simulink model "uz_SVPWM_6ph"  (R2024a)
settings: Solver=FixedStepDiscrete  StartTime=0.0  StopTime=0.0004  RelTol=1e-3
values from neighbouring files (symbols this model uses):
  f_FPGA_clk = 100e6    (= 100000000)    [Init_IP_Core.m]
  T_FPGA_clk = 1/f_FPGA_clk    (= 1e-08)    [Init_IP_Core.m]
libraries: hdlsllib x7, simulink x1
settings Model: DataTypeOverride=Off  Creator=josef  LastModifiedBy=josef
settings SolverCC: AlgebraicLoopSolver=TrustRegion
settings DataIOCC: LimitDataPoints=on  SaveOutput=off  SaveTime=off
settings OptimizationCC: BlockReduction=off  ConditionallyExecuteInputs=off  DefaultParameterBehavior=Inlined  LifeSpan=inf
settings DebuggingCC: AlgebraicLoopMsg=error  SingleTaskRateTransMsg=error  UnconnectedInputMsg=warning  UnconnectedOutputMsg=warning  UnconnectedLineMsg=warning  AllowSymbolicDim=off  StrictBusMsg=ErrorOnBusTreatedAsVector  SFUnexpectedBacktrackingDiag=warning  SFNoUnconditionalDefaultTransitionDiag=warning  SFExecutionAtInitializationDiag=none  ArithmeticOperatorsInVariantConditions=warning
settings HardwareCC: ProdBitPerPointer=32  ProdBitPerSizeT=32  ProdBitPerPtrDiffT=32  ProdLargestAtomicFloat=None  ProdIntDivRoundTo=Undefined  ProdEndianess=Unspecified  ProdWordSize=32  ProdHWDeviceType=ASIC/FPGA->ASIC/FPGA  ProdEqTarget=off
settings ModelReferenceCC: EnableRefExpFcnMdlSchedulingChecks=on
settings SFSimCC: SimUseLocalCustomCode=off  CustomCodeUndefinedFunction=UseInterfaceOnly
settings RTWCC: RTWUseLocalCustomCode=off  GPUComputeCapability=3.5
settings CodeAppCC: StateflowObjectComments=on
settings GRTTargetCC: TargetLangStandard=C89/C90 (ANSI)
settings ConfigComp: CovScope=ReferencedModels  CovMetricSettings=dw  CovSaveCumulativeToWorkspaceVar=on  CovSaveSingleToWorkspaceVar=on  CovExternalEMLEnable=off  CovSFcnEnable=off

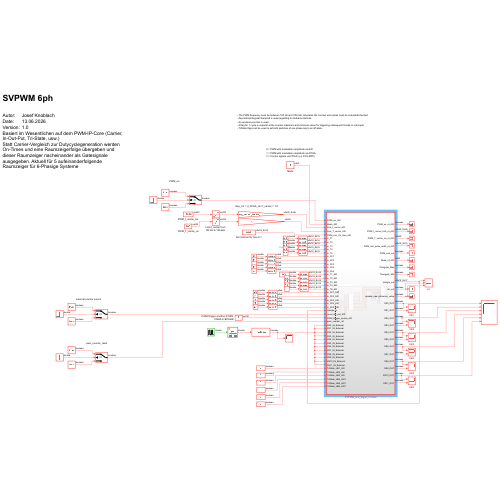
[thumbnail: Simulink's stored preview of the top-level diagram]
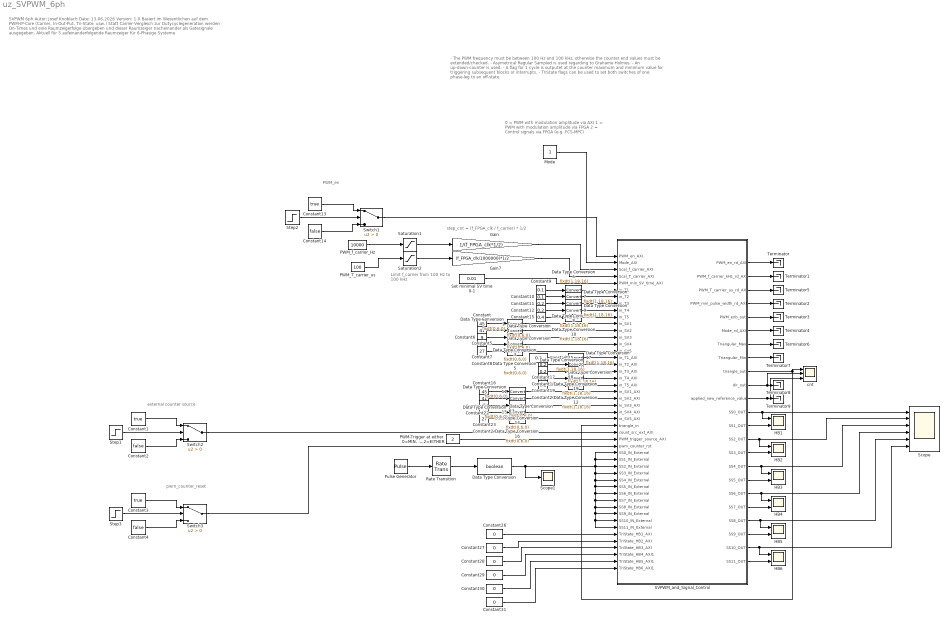
== system uz_SVPWM_6ph ==
  note: PWM_en
  note: Limit f_carrier from
      | 100 Hz to 100 kHz
  note: - The PWM frequency must be between 100 Hz and 100 kHz, otherwise the counter end values must be extended/checked.
      | - Asymetrical Regular Sampled is used regarding to Grahame Holmes.
      | - An up-down-counter is used.
      | - A flag for 1 cycle is outputet at the counter maximum and minimum value for triggering subsequent blocks or interrupts.
      | - TriState flags can be used to set both switches of one phase-leg to an off-state.
  note: SVPWM 6ph
      |
      | Autor: Josef Knoblach
      | Date: 13.06.2026
      | Version: 1.0
      | Basiert im Wesentlichen auf dem PWM-IP-Core (Carrier, In-Out-Put, Tri-State, usw.)
      | Statt Carrier-Vergleich zur Dutycyclegeneration werden On-Times und eine Raumzeigerfolge übergeben und dieser Raumzeiger nacheinander als Gatesignale ausgegeben. Aktuell für 5 aufeinanderfolgende Raumzeiger für 6-Phasige Systeme
  note: step_cnt = (f_FPGA_clk / f_carrier) * 1/2
  note: 0 = PWM with modulation amplitude via AXI
      | 1 = PWM with modulation amplitude via FPGA
      | 2 = Control signals via FPGA (e.g. FCS-MPC)
  note: external counter source
  note: pwm_counter_reset
  Constant : Constant  Value=45  SampleTime=T_FPGA_clk
  Constant1 : Constant  Value=true  SampleTime=T_FPGA_clk
  Constant10 : Constant  Value=0.1  SampleTime=T_FPGA_clk
  Constant{11..12,17..18,20} (5 alike) : Constant  Value=0.2  SampleTime=T_FPGA_clk
  Constant13 : Constant  Value=true  SampleTime=T_FPGA_clk
  Constant14 : Constant  Value=false  SampleTime=T_FPGA_clk
  Constant15 : Constant  Value=0.4  SampleTime=T_FPGA_clk
  Constant16 : Constant  Value=45  SampleTime=T_FPGA_clk
  Constant19 : Constant  Value=0.1  SampleTime=T_FPGA_clk
  Constant2 : Constant  Value=false  SampleTime=T_FPGA_clk
  Constant21 : Constant  Value=41  SampleTime=T_FPGA_clk
  Constant22 : Constant  Value=9  SampleTime=T_FPGA_clk
  Constant23 : Constant  Value=11  SampleTime=T_FPGA_clk
  Constant24 : Constant  Value=27  SampleTime=T_FPGA_clk
  Constant25 : Constant  Value=0.3  SampleTime=T_FPGA_clk
  Constant{26..31} (6 alike) : Constant  Value=0  OutDataTypeStr=boolean  SampleTime=T_FPGA_clk
  Constant3 : Constant  Value=true  SampleTime=T_FPGA_clk
  Constant4 : Constant  Value=false  SampleTime=T_FPGA_clk
  Constant5 : Constant  Value=41  SampleTime=T_FPGA_clk
  Constant6 : Constant  Value=9  SampleTime=T_FPGA_clk
  Constant7 : Constant  Value=11  SampleTime=T_FPGA_clk
  Constant8 : Constant  Value=27  SampleTime=T_FPGA_clk
  Constant9 : Constant  Value=0.1  SampleTime=T_FPGA_clk
  Data Type Conversion : DataTypeConversion  OutDataTypeStr=boolean  SaturateOnIntegerOverflow=off  RndMeth=Floor
  Data Type Conversion{1..5,11,13..16} (10 alike) : DataTypeConversion  OutDataTypeStr=fixdt(0,6,0)  SaturateOnIntegerOverflow=off  RndMeth=Floor
  Data Type Conversion{6..10,12,17..20} (10 alike) : DataTypeConversion  OutDataTypeStr=fixdt(1,18,16)  SaturateOnIntegerOverflow=off  RndMeth=Floor
  Gain : Gain  Gain=1/(f_FPGA_clk*1/2)  OutDataTypeStr=fixdt(0,25,26)
  Gain7 : Gain  Gain=(f_FPGA_clk/1000000)*1/2  OutDataTypeStr=fixdt(0,25,0)
  HB{1..6} (6 alike) : Scope  NumInputPorts=2
  Mode : Constant  OutDataTypeStr=fixdt(0,2,0)  SampleTime=T_FPGA_clk
  "PWM-Trigger at either 0=MIN, 1=MAX,2=EITHER" : Constant  Value=2  OutDataTypeStr=uint32  SampleTime=T_FPGA_clk
  PWM_T_carrier_us : Constant  Value=100  OutDataTypeStr=uint32  SampleTime=T_FPGA_clk
  PWM_f_carrier_Hz : Constant  Value=10000  OutDataTypeStr=uint32  SampleTime=T_FPGA_clk
  Pulse Generator : DiscretePulseGenerator  PulseType=Time based  Period=0.0001  PulseWidth=5
  Rate Transition : RateTransition  OutPortSampleTime=T_FPGA_clk
  SVPWM_and_Signal_Control : Subsystem  TreatAsAtomicUnit=on
  Saturation1 : Saturate  UpperLimit=100000  LowerLimit=100
  Saturation2 : Saturate  UpperLimit=10000  LowerLimit=10
  Scope : Scope  NumInputPorts=6
  Scope1 : Scope
  Set minimal SV time 0-1 : Constant  Value=0.01  OutDataTypeStr=fixdt(1,18,16)  SampleTime=T_FPGA_clk
  Step1 : Step  Time=0.002  After=0  SampleTime=T_FPGA_clk
  Step2 : Step  Time=0.002  Before=1  SampleTime=T_FPGA_clk
  Step3 : Step  Time=0.00025  SampleTime=T_FPGA_clk
  Switch1 : Switch  Criteria=u2 > Threshold  SaturateOnIntegerOverflow=off  InputSameDT=off
  Switch2 : Switch  Criteria=u2 > Threshold  SaturateOnIntegerOverflow=off  InputSameDT=off
  Switch3 : Switch  Criteria=u2 > Threshold  SaturateOnIntegerOverflow=off  InputSameDT=off
  Terminator{,1..9} (10 alike) : Terminator
  cnt : Scope  NumInputPorts=3
  wires:
  SVPWM_and_Signal_Control/9(triangle_out) -> SVPWM_and_Signal_Control/26(triangle_in), cnt/1
  Constant3/1 -> Switch3/1
  Pulse Generator/1 -> Rate Transition/1
  SVPWM_and_Signal_Control/11(applied_new_reference_value) -> cnt/3, Terminator9/1
  Constant4/1 -> Switch3/3
  Switch1/1 -> SVPWM_and_Signal_Control/1(PWM_en_AXI)
  SVPWM_and_Signal_Control/1(PWM_en_rd_AXI) -> Terminator/1
  Step3/1 -> Switch3/2
  "PWM-Trigger at either 0=MIN, 1=MAX,2=EITHER"/1 -> SVPWM_and_Signal_Control/28(PWM_trigger_source_AXI)
  SVPWM_and_Signal_Control/3(PWM_T_carrier_us_rd_AXI) -> Terminator5/1
  Switch3/1 -> SVPWM_and_Signal_Control/29(pwm_counter_rst)
  Switch2/1 -> SVPWM_and_Signal_Control/27(count_src_ext_AXI)
  SVPWM_and_Signal_Control/4(PWM_min_pulse_width_rd_AXI) -> Terminator2/1
  Rate Transition/1 -> Data Type Conversion/1
  PWM_T_carrier_us/1 -> Saturation2/1
  Step1/1 -> Switch2/2
  Saturation2/1 -> Gain7/1
  Saturation1/1 -> Gain/1
  Constant2/1 -> Switch2/3
  Constant14/1 -> Switch1/3
  SVPWM_and_Signal_Control/10(dir_out) -> cnt/2, Terminator8/1
  Constant1/1 -> Switch2/1
  SVPWM_and_Signal_Control/7(Triangular_Max) -> Terminator6/1
  SVPWM_and_Signal_Control/2(PWM_f_carrier_kHz_rd_AXI) -> Terminator1/1
  SVPWM_and_Signal_Control/5(PWM_enb_out) -> Terminator3/1
  Gain7/1 -> SVPWM_and_Signal_Control/4(Scal_T_carrier_AXI)
  SVPWM_and_Signal_Control/6(Mode_rd_AXI) -> Terminator4/1
  Gain/1 -> SVPWM_and_Signal_Control/3(Scal_f_carrier_AXI)
  SVPWM_and_Signal_Control/8(Triangular_Min) -> Terminator7/1
  Step2/1 -> Switch1/2
  Set minimal SV time 0-1/1 -> SVPWM_and_Signal_Control/5(PWM_min_SV_time_AXI)
  Mode/1 -> SVPWM_and_Signal_Control/2(Mode_AXI)
  PWM_f_carrier_Hz/1 -> Saturation1/1
  Constant13/1 -> Switch1/1
  Data Type Conversion5/1 -> SVPWM_and_Signal_Control/15(in_SV5)
  Data Type Conversion4/1 -> SVPWM_and_Signal_Control/14(in_SV4)
  Data Type Conversion3/1 -> SVPWM_and_Signal_Control/13(in_SV3)
  Data Type Conversion2/1 -> SVPWM_and_Signal_Control/12(in_SV2)
  Data Type Conversion1/1 -> SVPWM_and_Signal_Control/11(in_SV1)
  Constant/1 -> Data Type Conversion1/1
  Constant8/1 -> Data Type Conversion5/1
  Constant7/1 -> Data Type Conversion4/1
  Constant6/1 -> Data Type Conversion3/1
  Constant5/1 -> Data Type Conversion2/1
  Constant10/1 -> Data Type Conversion7/1
  Constant11/1 -> Data Type Conversion8/1
  Constant12/1 -> Data Type Conversion9/1
  Constant15/1 -> Data Type Conversion10/1
  Constant9/1 -> Data Type Conversion6/1
  Data Type Conversion6/1 -> SVPWM_and_Signal_Control/6(in_T1)
  Data Type Conversion10/1 -> SVPWM_and_Signal_Control/10(in_T5)
  Data Type Conversion9/1 -> SVPWM_and_Signal_Control/9(in_T4)
  Data Type Conversion8/1 -> SVPWM_and_Signal_Control/8(in_T3)
  Data Type Conversion7/1 -> SVPWM_and_Signal_Control/7(in_T2)
  Data Type Conversion18/1 -> SVPWM_and_Signal_Control/17(in_T2_AXI)
  Data Type Conversion19/1 -> SVPWM_and_Signal_Control/18(in_T3_AXI)
  Data Type Conversion20/1 -> SVPWM_and_Signal_Control/19(in_T4_AXI)
  Data Type Conversion12/1 -> SVPWM_and_Signal_Control/20(in_T5_AXI)
  Data Type Conversion17/1 -> SVPWM_and_Signal_Control/16(in_T1_AXI)
  Constant25/1 -> Data Type Conversion17/1
  Constant20/1 -> Data Type Conversion12/1
  Constant19/1 -> Data Type Conversion20/1
  Constant18/1 -> Data Type Conversion19/1
  Constant17/1 -> Data Type Conversion18/1
  Constant21/1 -> Data Type Conversion13/1
  Constant22/1 -> Data Type Conversion14/1
  Constant23/1 -> Data Type Conversion15/1
  Constant24/1 -> Data Type Conversion16/1
  Constant16/1 -> Data Type Conversion11/1
  Data Type Conversion11/1 -> SVPWM_and_Signal_Control/21(in_SV1_AXI)
  Data Type Conversion13/1 -> SVPWM_and_Signal_Control/22(in_SV2_AXI)
  Data Type Conversion14/1 -> SVPWM_and_Signal_Control/23(in_SV3_AXI)
  Data Type Conversion15/1 -> SVPWM_and_Signal_Control/24(in_SV4_AXI)
  Data Type Conversion16/1 -> SVPWM_and_Signal_Control/25(in_SV5_AXI)
  Data Type Conversion/1 -> Scope1/1, SVPWM_and_Signal_Control/41(SS11_IN_External), SVPWM_and_Signal_Control/40(SS10_IN_External), SVPWM_and_Signal_Control/39(SS9_IN_External), SVPWM_and_Signal_Control/38(SS8_IN_External), SVPWM_and_Signal_Control/37(SS7_IN_External), SVPWM_and_Signal_Control/36(SS6_IN_External), SVPWM_and_Signal_Control/35(SS5_IN_External), SVPWM_and_Signal_Control/34(SS4_IN_External), SVPWM_and_Signal_Control/33(SS3_IN_External), SVPWM_and_Signal_Control/32(SS2_IN_External), SVPWM_and_Signal_Control/31(SS1_IN_External), SVPWM_and_Signal_Control/30(SS0_IN_External)
  Constant26/1 -> SVPWM_and_Signal_Control/42(TriState_HB1_AXI)
  Constant27/1 -> SVPWM_and_Signal_Control/43(TriState_HB2_AXI)
  Constant28/1 -> SVPWM_and_Signal_Control/44(TriState_HB3_AXI)
  Constant29/1 -> SVPWM_and_Signal_Control/45(TriState_HB4_AXI1)
  Constant30/1 -> SVPWM_and_Signal_Control/46(TriState_HB5_AXI1)
  Constant31/1 -> SVPWM_and_Signal_Control/47(TriState_HB6_AXI1)
  SVPWM_and_Signal_Control/12(SS0_OUT) -> HB1/1, Scope/1
  SVPWM_and_Signal_Control/14(SS2_OUT) -> HB2/1, Scope/2
  SVPWM_and_Signal_Control/16(SS4_OUT) -> HB3/1, Scope/3
  SVPWM_and_Signal_Control/18(SS6_OUT) -> HB4/1, Scope/4
  SVPWM_and_Signal_Control/20(SS8_OUT) -> HB5/1, Scope/5
  SVPWM_and_Signal_Control/22(SS10_OUT) -> HB6/1, Scope/6
  SVPWM_and_Signal_Control/13(SS1_OUT) -> HB1/2
  SVPWM_and_Signal_Control/23(SS11_OUT) -> HB6/2
  SVPWM_and_Signal_Control/21(SS9_OUT) -> HB5/2
  SVPWM_and_Signal_Control/19(SS7_OUT) -> HB4/2
  SVPWM_and_Signal_Control/17(SS5_OUT) -> HB3/2
  SVPWM_and_Signal_Control/15(SS3_OUT) -> HB2/2

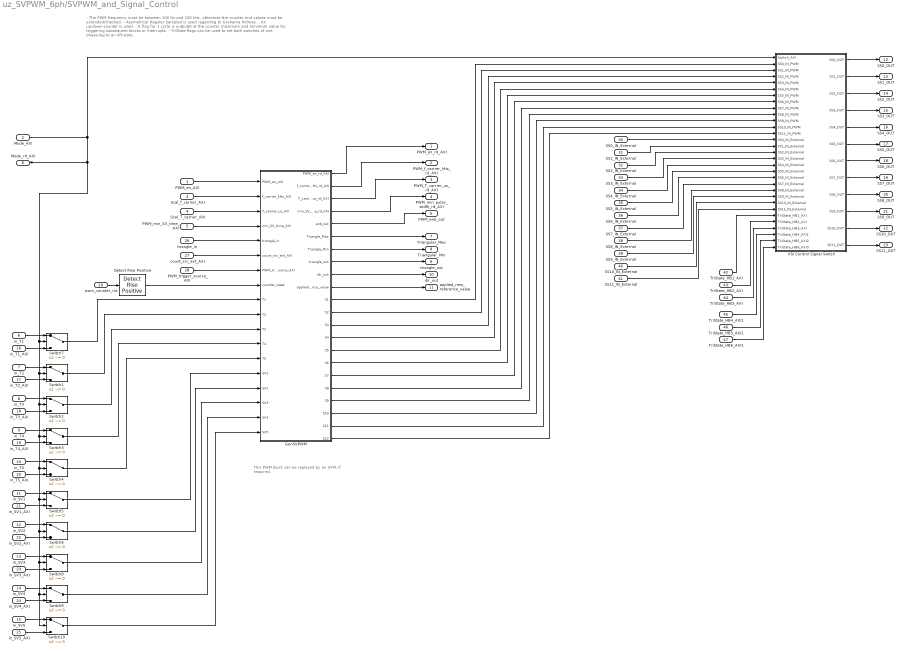
== system uz_SVPWM_6ph/SVPWM_and_Signal_Control ==
  note: This PWM block can be replaced by an SVM,
      | if required.
  note: - The PWM frequency must be between 100 Hz and 100 kHz, otherwise the counter end values must be extended/checked.
      | - Asymetrical Regular Sampled is used regarding to Grahame Holmes.
      | - An up-down-counter is used.
      | - A flag for 1 cycle is outputet at the counter maximum and minimum value for triggering subsequent blocks or interrupts.
      | - TriState flags can be used to set both switches of one phase-leg to an off-state.
  PWM_en_AXI : Inport
  Mode_AXI : Inport  Port=2
  Scal_f_carrier_AXI : Inport  Port=3
  Scal_T_carrier_AXI : Inport  Port=4
  PWM_min_SV_time_AXI : Inport  Port=5
  in_T1 : Inport  Port=6
  in_T2 : Inport  Port=7
  in_T3 : Inport  Port=8
  in_T4 : Inport  Port=9
  in_T5 : Inport  Port=10
  in_SV1 : Inport  Port=11
  in_SV2 : Inport  Port=12
  in_SV3 : Inport  Port=13
  in_SV4 : Inport  Port=14
  in_SV5 : Inport  Port=15
  in_T1_AXI : Inport  Port=16
  in_T2_AXI : Inport  Port=17
  in_T3_AXI : Inport  Port=18
  in_T4_AXI : Inport  Port=19
  in_T5_AXI : Inport  Port=20
  in_SV1_AXI : Inport  Port=21
  in_SV2_AXI : Inport  Port=22
  in_SV3_AXI : Inport  Port=23
  in_SV4_AXI : Inport  Port=24
  in_SV5_AXI : Inport  Port=25
  triangle_in : Inport  Port=26
  count_src_ext_AXI : Inport  Port=27
  PWM_trigger_source_AXI : Inport  Port=28
  pwm_counter_rst : Inport  Port=29
  SS0_IN_External : Inport  Port=30
  SS1_IN_External : Inport  Port=31
  SS2_IN_External : Inport  Port=32
  SS3_IN_External : Inport  Port=33
  SS4_IN_External : Inport  Port=34
  SS5_IN_External : Inport  Port=35
  SS6_IN_External : Inport  Port=36
  SS7_IN_External : Inport  Port=37
  SS8_IN_External : Inport  Port=38
  SS9_IN_External : Inport  Port=39
  SS10_IN_External : Inport  Port=40
  SS11_IN_External : Inport  Port=41
  TriState_HB1_AXI : Inport  Port=42
  TriState_HB2_AXI : Inport  Port=43
  TriState_HB3_AXI : Inport  Port=44
  TriState_HB4_AXI1 : Inport  Port=45
  TriState_HB5_AXI1 : Inport  Port=46
  TriState_HB6_AXI1 : Inport  Port=47
  Detect Rise Positive : simulink/Logic and Bit Operations/Detect Rise Positive  vinit=0  OutDataTypeStr=boolean
  GenSVPWM : Subsystem  TreatAsAtomicUnit=on
  Switch{1..10} (10 alike) : Switch  Criteria=u2 ~= 0  SaturateOnIntegerOverflow=off  InputSameDT=off
  VSI Control Signal Switch : Subsystem
  PWM_en_rd_AXI : Outport  VectorParamsAs1DForOutWhenUnconnected=off
  PWM_f_carrier_kHz_rd_AXI : Outport  Port=2  VectorParamsAs1DForOutWhenUnconnected=off
  PWM_T_carrier_us_rd_AXI : Outport  Port=3  VectorParamsAs1DForOutWhenUnconnected=off
  PWM_min_pulse_width_rd_AXI : Outport  Port=4  VectorParamsAs1DForOutWhenUnconnected=off
  PWM_enb_out : Outport  Port=5  VectorParamsAs1DForOutWhenUnconnected=off
  Mode_rd_AXI : Outport  Port=6  VectorParamsAs1DForOutWhenUnconnected=off
  Triangular_Max : Outport  Port=7  VectorParamsAs1DForOutWhenUnconnected=off
  Triangular_Min : Outport  Port=8  VectorParamsAs1DForOutWhenUnconnected=off
  triangle_out : Outport  Port=9  VectorParamsAs1DForOutWhenUnconnected=off
  dir_out : Outport  Port=10  VectorParamsAs1DForOutWhenUnconnected=off
  applied_new_reference_value : Outport  Port=11  VectorParamsAs1DForOutWhenUnconnected=off
  SS0_OUT : Outport  Port=12  VectorParamsAs1DForOutWhenUnconnected=off
  SS1_OUT : Outport  Port=13  VectorParamsAs1DForOutWhenUnconnected=off
  SS2_OUT : Outport  Port=14  VectorParamsAs1DForOutWhenUnconnected=off
  SS3_OUT : Outport  Port=15  VectorParamsAs1DForOutWhenUnconnected=off
  SS4_OUT : Outport  Port=16  VectorParamsAs1DForOutWhenUnconnected=off
  SS5_OUT : Outport  Port=17  VectorParamsAs1DForOutWhenUnconnected=off
  SS6_OUT : Outport  Port=18  VectorParamsAs1DForOutWhenUnconnected=off
  SS7_OUT : Outport  Port=19  VectorParamsAs1DForOutWhenUnconnected=off
  SS8_OUT : Outport  Port=20  VectorParamsAs1DForOutWhenUnconnected=off
  SS9_OUT : Outport  Port=21  VectorParamsAs1DForOutWhenUnconnected=off
  SS10_OUT : Outport  Port=22  VectorParamsAs1DForOutWhenUnconnected=off
  SS11_OUT : Outport  Port=23  VectorParamsAs1DForOutWhenUnconnected=off
  wires:
  Scal_f_carrier_AXI/1 -> GenSVPWM/2(f_carrier_kHz_AXI)
  GenSVPWM/5(enb_out) -> PWM_enb_out/1
  PWM_en_AXI/1 -> GenSVPWM/1(PWM_en_AXI)
  PWM_min_SV_time_AXI/1 -> GenSVPWM/4(min_SV_time_AXI)
  in_T1_AXI/1 -> Switch7/3
  in_T1/1 -> Switch7/1
  GenSVPWM/1(PWM_en_rd_AXI) -> PWM_en_rd_AXI/1
  GenSVPWM/2(f_carrier_kHz_rd_AXI) -> PWM_f_carrier_kHz_rd_AXI/1
  GenSVPWM/4(min_SV_time_rd_AXI) -> PWM_min_pulse_width_rd_AXI/1
  GenSVPWM/3(T_carrier_us_rd_AXI) -> PWM_T_carrier_us_rd_AXI/1
  Scal_T_carrier_AXI/1 -> GenSVPWM/3(T_carrier_us_AXI)
  GenSVPWM/6(Triangle_Max) -> Triangular_Max/1
  GenSVPWM/7(Triangle_Min) -> Triangular_Min/1
  triangle_in/1 -> GenSVPWM/5(triangle_in)
  GenSVPWM/8(triangle_out) -> triangle_out/1
  GenSVPWM/9(dir_out) -> dir_out/1
  count_src_ext_AXI/1 -> GenSVPWM/6(count_src_ext_AXI)
  PWM_trigger_source_AXI/1 -> GenSVPWM/7(PWM_trigger_source_AXI)
  GenSVPWM/10(applied_new_reference_value) -> applied_new_reference_value/1
  Detect Rise Positive/1 -> GenSVPWM/8(counter_reset)
  pwm_counter_rst/1 -> Detect Rise Positive/1
  VSI Control Signal Switch/8(SS7_OUT) -> SS7_OUT/1
  SS10_IN_External/1 -> VSI Control Signal Switch/24(SS10_IN_External)
  SS8_IN_External/1 -> VSI Control Signal Switch/22(SS8_IN_External)
  SS6_IN_External/1 -> VSI Control Signal Switch/20(SS6_IN_External)
  TriState_HB4_AXI1/1 -> VSI Control Signal Switch/29(TriState_HB4_AXI1)
  TriState_HB2_AXI/1 -> VSI Control Signal Switch/27(TriState_HB2_AXI)
  SS9_IN_External/1 -> VSI Control Signal Switch/23(SS9_IN_External)
  TriState_HB3_AXI/1 -> VSI Control Signal Switch/28(TriState_HB3_AXI)
  VSI Control Signal Switch/10(SS9_OUT) -> SS9_OUT/1
  TriState_HB1_AXI/1 -> VSI Control Signal Switch/26(TriState_HB1_AXI)
  VSI Control Signal Switch/5(SS4_OUT) -> SS4_OUT/1
  VSI Control Signal Switch/1(SS0_OUT) -> SS0_OUT/1
  SS7_IN_External/1 -> VSI Control Signal Switch/21(SS7_IN_External)
  VSI Control Signal Switch/6(SS5_OUT) -> SS5_OUT/1
  SS1_IN_External/1 -> VSI Control Signal Switch/15(SS1_IN_External)
  SS4_IN_External/1 -> VSI Control Signal Switch/18(SS4_IN_External)
  SS3_IN_External/1 -> VSI Control Signal Switch/17(SS3_IN_External)
  SS5_IN_External/1 -> VSI Control Signal Switch/19(SS5_IN_External)
  VSI Control Signal Switch/4(SS3_OUT) -> SS3_OUT/1
  VSI Control Signal Switch/2(SS1_OUT) -> SS1_OUT/1
  SS2_IN_External/1 -> VSI Control Signal Switch/16(SS2_IN_External)
  VSI Control Signal Switch/3(SS2_OUT) -> SS2_OUT/1
  VSI Control Signal Switch/9(SS8_OUT) -> SS8_OUT/1
  VSI Control Signal Switch/12(SS11_OUT) -> SS11_OUT/1
  VSI Control Signal Switch/11(SS10_OUT) -> SS10_OUT/1
  Mode_AXI/1 -> Mode_rd_AXI/1, Switch10/2, Switch9/2, Switch8/2, Switch6/2, Switch5/2, Switch4/2, Switch3/2, Switch2/2, Switch1/2, Switch7/2, VSI Control Signal Switch/1(Switch_AXI)
  SS11_IN_External/1 -> VSI Control Signal Switch/25(SS11_IN_External)
  TriState_HB6_AXI1/1 -> VSI Control Signal Switch/31(TriState_HB6_AXI3)
  VSI Control Signal Switch/7(SS6_OUT) -> SS6_OUT/1
  TriState_HB5_AXI1/1 -> VSI Control Signal Switch/30(TriState_HB5_AXI2)
  SS0_IN_External/1 -> VSI Control Signal Switch/14(SS0_IN_External)
  GenSVPWM/11(S1) -> VSI Control Signal Switch/2(SS0_IN_PWM)
  GenSVPWM/12(S2) -> VSI Control Signal Switch/3(SS1_IN_PWM)
  GenSVPWM/13(S3) -> VSI Control Signal Switch/4(SS2_IN_PWM)
  GenSVPWM/14(S4) -> VSI Control Signal Switch/5(SS3_IN_PWM)
  GenSVPWM/15(S5) -> VSI Control Signal Switch/6(SS4_IN_PWM)
  GenSVPWM/16(S6) -> VSI Control Signal Switch/7(SS5_IN_PWM)
  GenSVPWM/17(S7) -> VSI Control Signal Switch/8(SS6_IN_PWM)
  GenSVPWM/18(S8) -> VSI Control Signal Switch/9(SS7_IN_PWM)
  GenSVPWM/19(S9) -> VSI Control Signal Switch/10(SS8_IN_PWM)
  GenSVPWM/20(S10) -> VSI Control Signal Switch/11(SS9_IN_PWM)
  GenSVPWM/21(S11) -> VSI Control Signal Switch/12(SS10_IN_PWM)
  GenSVPWM/22(S12) -> VSI Control Signal Switch/13(SS11_IN_PWM)
  in_T2/1 -> Switch1/1
  in_T2_AXI/1 -> Switch1/3
  in_T3/1 -> Switch2/1
  in_T3_AXI/1 -> Switch2/3
  in_T4/1 -> Switch3/1
  in_T4_AXI/1 -> Switch3/3
  in_T5/1 -> Switch4/1
  in_T5_AXI/1 -> Switch4/3
  in_SV1/1 -> Switch5/1
  in_SV1_AXI/1 -> Switch5/3
  in_SV2/1 -> Switch6/1
  in_SV2_AXI/1 -> Switch6/3
  in_SV3/1 -> Switch8/1
  in_SV3_AXI/1 -> Switch8/3
  in_SV4_AXI/1 -> Switch9/3
  in_SV4/1 -> Switch9/1
  in_SV5_AXI/1 -> Switch10/3
  in_SV5/1 -> Switch10/1
  Switch7/1 -> GenSVPWM/9(T1)
  Switch1/1 -> GenSVPWM/10(T2)
  Switch2/1 -> GenSVPWM/11(T3)
  Switch3/1 -> GenSVPWM/12(T4)
  Switch4/1 -> GenSVPWM/13(T5)
  Switch5/1 -> GenSVPWM/14(SV1)
  Switch6/1 -> GenSVPWM/15(SV2)
  Switch8/1 -> GenSVPWM/16(SV3)
  Switch9/1 -> GenSVPWM/17(SV4)
  Switch10/1 -> GenSVPWM/18(SV5)

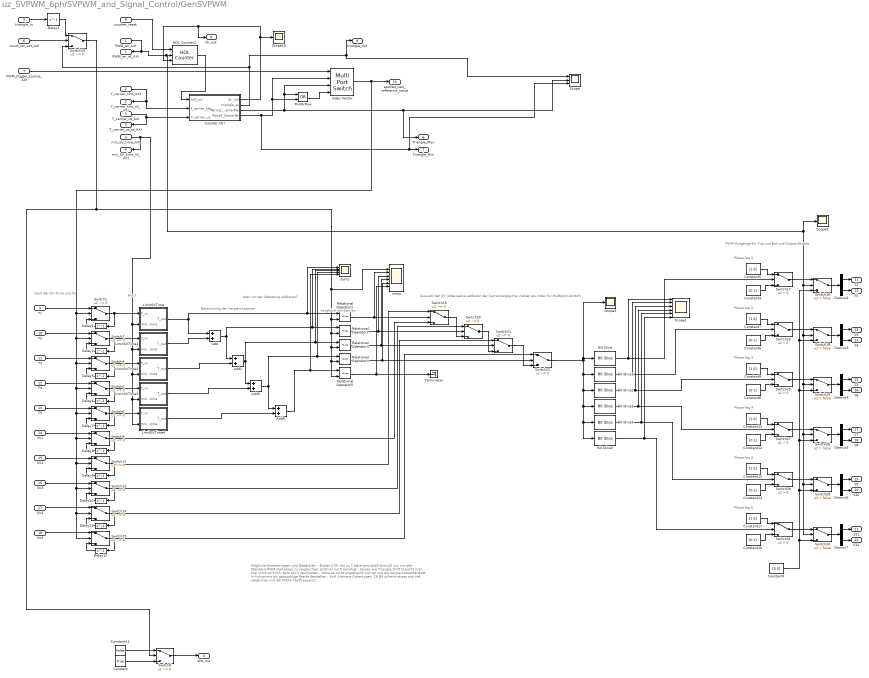
== system uz_SVPWM_6ph/SVPWM_and_Signal_Control/GenSVPWM ==
  note: Min T
  note: PWM-Ausgänge für Top und Bot und Output-Enable
  note: Auswahl der SV
      | (Alternative addieren der Carriervergleiche, nutzen als index für Multiport-Switch)
  note: Mögliche Erweiterungen und Gedanken:
      | - Bisher 5 SV, bis zu 7 wäre prinzipiell sinnvoll um mit den Standard-PWM-Verfahren zu vergleichen, erstmal nur 5 benötigt
      | - Sowas wie Triangle-Shift braucht man hier nicht wirklich, falls doch nachrüsten
      | - Wäre es nicht angebracht Carrier und die Vergleichswerte statt in fixkomma als ganzzahlige Werte darstellen
      | - Evtl. kleinere Datentypen, 18 Bit scheint etwas arg viel verglichen mit der FPGA-Taktfrequenz?
  note: Vergleich mit Carrier
  note: Berechnung der Vergleichszeiten
  note: Input der On-Time und SV
  note: oder vor der Abtastung addieren?
  note: Phase-leg 1
  note: Phase-leg 2
  note: Phase-leg 3
  note: Phase-leg 4
  note: Phase-leg 5
  note: Phase-leg 6
  PWM_en_AXI : Inport
  f_carrier_kHz_AXI : Inport  Port=2
  T_carrier_us_AXI : Inport  Port=3
  min_SV_time_AXI : Inport  Port=4
  triangle_in : Inport  Port=5
  count_src_ext_AXI : Inport  Port=6
  PWM_trigger_source_AXI : Inport  Port=7
  counter_reset : Inport  Port=8
  T1 : Inport  Port=9
  T2 : Inport  Port=10
  T3 : Inport  Port=11
  T4 : Inport  Port=12
  T5 : Inport  Port=13
  SV1 : Inport  Port=14
  SV2 : Inport  Port=15
  SV3 : Inport  Port=16
  SV4 : Inport  Port=17
  SV5 : Inport  Port=18
  Add{,2..4} (4 alike) : Sum
  Bit Slice : hdlsllib/Logic and Bit Operations/Bit Slice  lidx=0  ridx=0
  Bit Slice1 : hdlsllib/Logic and Bit Operations/Bit Slice  lidx=1  ridx=1
  Bit Slice2 : hdlsllib/Logic and Bit Operations/Bit Slice  lidx=2  ridx=2
  Bit Slice3 : hdlsllib/Logic and Bit Operations/Bit Slice  lidx=3  ridx=3
  Bit Slice4 : hdlsllib/Logic and Bit Operations/Bit Slice  lidx=4  ridx=4
  Bit Slice5 : hdlsllib/Logic and Bit Operations/Bit Slice  lidx=5  ridx=5
  Constant : Constant  Value=true  SampleTime=T_FPGA_clk
  Constant11 : Constant  Value=false  SampleTime=T_FPGA_clk
  Constant{3,6,8,12,14,16} (6 alike) : Constant  Value=[0 1]  OutDataTypeStr=fixdt(0,1,0)  SampleTime=T_FPGA_clk
  Constant{5,7,9,13,15,17} (6 alike) : Constant  Value=[1 0]  OutDataTypeStr=fixdt(0,1,0)  SampleTime=T_FPGA_clk
  Constant4 : Constant  Value=[0 0]  OutDataTypeStr=fixdt(0,1,0)  SampleTime=T_FPGA_clk
  Counter Ctrl : Subsystem
  Delay{1..2,4..12} (11 alike) : Delay  DelayLength=1
  Demux{2..7} (6 alike) : Demux  Outputs=2
  HDL Counter2 : hdlsllib/Sources/HDL Counter  CountType=Free running  CountInit=0  CountStep=1  CountMax=100  CountFromType=Initial value  CountFrom=0  CountResetPort=on  CountLoadPort=off  CountEnbPort=on  CountDirPort=on  CountHitOutputPort=off  CountDataType=Unsigned  CountWordLen=20  CountFracLen=0  CountSampTime=1
  Index Vector : MultiPortSwitch  DataPortOrder=Zero-based contiguous  zeroidx=on  SaturateOnIntegerOverflow=off  InputSameDT=off
  LimitSVTime : Subsystem
  LimitSVTime1 : Subsystem
  LimitSVTime2 : Subsystem
  LimitSVTime3 : Subsystem
  LimitSVTime4 : Subsystem
  MinOrMax : Logic  Operator=OR  AllPortsSameDT=off  OutDataTypeStr=boolean
  Relational Operator{1..5} (5 alike) : RelationalOperator  Operator=<=  OutDataTypeStr=boolean  InputSameDT=off
  Scope : Scope  NumInputPorts=3
  Scope1 : Scope  NumInputPorts=6
  Scope10 : Scope
  Scope2 : Scope
  Scope3 : Scope
  Sums : Scope  NumInputPorts=5
  Switch{1..2,4..5,8..10,12..15} (11 alike) : Switch  Criteria=u2 ~= 0  Threshold=1  SaturateOnIntegerOverflow=off  InputSameDT=off
  Switch{16,18,24,26,28,30} (6 alike) : Switch  Criteria=u2 > Threshold  Threshold=false  SaturateOnIntegerOverflow=off  InputSameDT=off
  Switch{17,23,25,27,29,31} (6 alike) : Switch  Criteria=u2 > Threshold  SaturateOnIntegerOverflow=off  InputSameDT=off
  Switch{6,19..22} (5 alike) : Switch  Criteria=u2 ~= 0  SaturateOnIntegerOverflow=off  InputSameDT=off
  Terminator : Terminator
  comp : Scope  NumInputPorts=6
  PWM_en_rd_AXI : Outport  VectorParamsAs1DForOutWhenUnconnected=off
  f_carrier_kHz_rd_AXI : Outport  Port=2  VectorParamsAs1DForOutWhenUnconnected=off
  T_carrier_us_rd_AXI : Outport  Port=3  VectorParamsAs1DForOutWhenUnconnected=off
  min_SV_time_rd_AXI : Outport  Port=4  VectorParamsAs1DForOutWhenUnconnected=off
  enb_out : Outport  Port=5  VectorParamsAs1DForOutWhenUnconnected=off
  Triangle_Max : Outport  Port=6  VectorParamsAs1DForOutWhenUnconnected=off
  Triangle_Min : Outport  Port=7  VectorParamsAs1DForOutWhenUnconnected=off
  triangle_out : Outport  Port=8  VectorParamsAs1DForOutWhenUnconnected=off
  dir_out : Outport  Port=9  VectorParamsAs1DForOutWhenUnconnected=off
  applied_new_reference_value : Outport  Port=10  OutDataTypeStr=boolean  VectorParamsAs1DForOutWhenUnconnected=off
  S1 : Outport  Port=11  VectorParamsAs1DForOutWhenUnconnected=off
  S2 : Outport  Port=12  VectorParamsAs1DForOutWhenUnconnected=off
  S3 : Outport  Port=13  VectorParamsAs1DForOutWhenUnconnected=off
  S4 : Outport  Port=14  VectorParamsAs1DForOutWhenUnconnected=off
  S5 : Outport  Port=15  VectorParamsAs1DForOutWhenUnconnected=off
  S6 : Outport  Port=16  VectorParamsAs1DForOutWhenUnconnected=off
  S7 : Outport  Port=17  VectorParamsAs1DForOutWhenUnconnected=off
  S8 : Outport  Port=18  VectorParamsAs1DForOutWhenUnconnected=off
  S9 : Outport  Port=19  VectorParamsAs1DForOutWhenUnconnected=off
  S10 : Outport  Port=20  VectorParamsAs1DForOutWhenUnconnected=off
  S11 : Outport  Port=21  VectorParamsAs1DForOutWhenUnconnected=off
  S12 : Outport  Port=22  VectorParamsAs1DForOutWhenUnconnected=off
  wires:
  Counter Ctrl/2(triangle_sig) -> triangle_out/1, Scope/1, Switch10/3
  PWM_en_AXI/1 -> Scope2/1, Switch30/2, Switch28/2, Switch26/2, Switch24/2, Switch18/2, Switch16/2, HDL Counter2/2, PWM_en_rd_AXI/1
  Counter Ctrl/1(dir_ctrl) -> dir_out/1, HDL Counter2/3, Scope10/1
  f_carrier_kHz_AXI/1 -> f_carrier_kHz_rd_AXI/1, Counter Ctrl/2(f_carrier_kHz)
  Switch6/1 -> enb_out/1
  Constant11/1 -> Switch6/1
  Constant/1 -> Switch6/3
  T_carrier_us_AXI/1 -> T_carrier_us_rd_AXI/1, Counter Ctrl/3(T_carrier_us)
  min_SV_time_AXI/1 -> LimitSVTime1/2(min_time), LimitSVTime2/2(min_time), LimitSVTime3/2(min_time), LimitSVTime4/2(min_time), LimitSVTime/2(min_time), min_SV_time_rd_AXI/1
  Counter Ctrl/3(Period_CenterMax) -> Index Vector/3, MinOrMax/1, Scope/2, Triangle_Max/1
  Counter Ctrl/4(Period_CenterMin) -> Scope/3, Triangle_Min/1, MinOrMax/2, Index Vector/2
  triangle_in/1 -> Delay4/1
  count_src_ext_AXI/1 -> Switch10/2
  HDL Counter2/1 -> Counter Ctrl/1(hdl_cnt)
  Delay4/1 -> Switch10/1
  Switch10/1 -> comp/1, Relational Operator5/2, Relational Operator4/2, Relational Operator3/2, Relational Operator2/2, Relational Operator1/2, Switch6/2
  MinOrMax/1 -> Index Vector/4
  PWM_trigger_source_AXI/1 -> Index Vector/1
  counter_reset/1 -> HDL Counter2/1
  Index Vector/1 -> applied_new_reference_value/1, Switch1/2, Switch13/2, Switch15/2, Switch14/2, Switch12/2, Switch9/2, Switch8/2, Switch5/2, Switch4/2, Switch2/2
  Switch1/1 -> LimitSVTime/1(T_in), Delay1/1
  Delay1/1 -> Switch1/3
  T1/1 -> Switch1/1
  T2/1 -> Switch2/1
  Delay2/1 -> Switch2/3
  Switch2/1 -> LimitSVTime1/1(T_in), Delay2/1
  Switch4/1 -> LimitSVTime2/1(T_in), Delay5/1
  Delay5/1 -> Switch4/3
  T3/1 -> Switch4/1
  T4/1 -> Switch5/1
  Delay6/1 -> Switch5/3
  Switch5/1 -> LimitSVTime3/1(T_in), Delay6/1
  Switch8/1 -> LimitSVTime4/1(T_in), Delay7/1
  Delay7/1 -> Switch8/3
  T5/1 -> Switch8/1
  SV1/1 -> Switch9/1
  Delay8/1 -> Switch9/3
  Switch9/1 -> Delay8/1, Switch19/3
  Switch12/1 -> Switch19/1, Delay9/1
  Delay9/1 -> Switch12/3
  SV2/1 -> Switch12/1
  SV3/1 -> Switch13/1
  Delay10/1 -> Switch13/3
  Switch13/1 -> Switch20/1, Delay10/1
  Switch14/1 -> Switch21/1, Delay11/1
  Delay11/1 -> Switch14/3
  SV4/1 -> Switch14/1
  SV5/1 -> Switch15/1
  Delay12/1 -> Switch15/3
  Switch15/1 -> Switch22/1, Delay12/1
  Relational Operator1/1 -> Switch19/2, comp/2
  Relational Operator2/1 -> Switch20/2, comp/3
  Relational Operator4/1 -> Switch22/2, comp/5
  Relational Operator5/1 -> Terminator/1, comp/6
  Relational Operator3/1 -> Switch21/2, comp/4
  Add/1 -> Sums/2, Relational Operator2/1, Add2/1
  Add2/1 -> Add3/1, Sums/3, Relational Operator3/1
  Add3/1 -> Sums/4, Relational Operator4/1, Add4/1
  Add4/1 -> Relational Operator5/1, Sums/5
  Switch19/1 -> Switch20/3
  Switch20/1 -> Switch21/3
  Switch21/1 -> Switch22/3
  Switch16/1 -> Demux2/1
  Bit Slice/1 -> Scope1/1, Switch17/2
  Switch17/1 -> Switch16/1
  Constant5/1 -> Switch17/1
  Constant3/1 -> Switch17/3
  Demux2/2 -> S2/1
  Demux2/1 -> S1/1
  Constant4/1 -> Switch16/3, Switch18/3, Switch24/3, Switch26/3, Switch28/3, Switch30/3
  Constant7/1 -> Switch23/1
  Constant6/1 -> Switch23/3
  Demux3/2 -> S4/1
  Demux3/1 -> S3/1
  Switch23/1 -> Switch18/1
  Bit Slice1/1 -> Scope1/2, Switch23/2
  Switch18/1 -> Demux3/1
  Constant9/1 -> Switch25/1
  Constant8/1 -> Switch25/3
  Demux4/2 -> S6/1
  Demux4/1 -> S5/1
  Switch25/1 -> Switch24/1
  Bit Slice2/1 -> Scope1/3, Switch25/2
  Switch24/1 -> Demux4/1
  Constant13/1 -> Switch27/1
  Constant12/1 -> Switch27/3
  Demux5/2 -> S8/1
  Demux5/1 -> S7/1
  Switch27/1 -> Switch26/1
  Bit Slice3/1 -> Scope1/4, Switch27/2
  Switch26/1 -> Demux5/1
  Constant15/1 -> Switch29/1
  Constant14/1 -> Switch29/3
  Demux6/2 -> S10/1
  Demux6/1 -> S9/1
  Switch29/1 -> Switch28/1
  Bit Slice4/1 -> Switch29/2, Scope1/5
  Switch28/1 -> Demux6/1
  Constant17/1 -> Switch31/1
  Constant16/1 -> Switch31/3
  Demux7/2 -> S12/1
  Demux7/1 -> S11/1
  Switch31/1 -> Switch30/1
  Bit Slice5/1 -> Scope1/6, Switch31/2
  Switch30/1 -> Demux7/1
  LimitSVTime/1(T_out) -> Add/1, Sums/1, Relational Operator1/1
  LimitSVTime1/1(T_out) -> Add/2
  LimitSVTime2/1(T_out) -> Add2/2
  LimitSVTime3/1(T_out) -> Add3/2
  LimitSVTime4/1(T_out) -> Add4/2
  Switch22/1 -> Bit Slice5/1, Bit Slice4/1, Bit Slice3/1, Bit Slice2/1, Bit Slice1/1, Scope3/1, Bit Slice/1

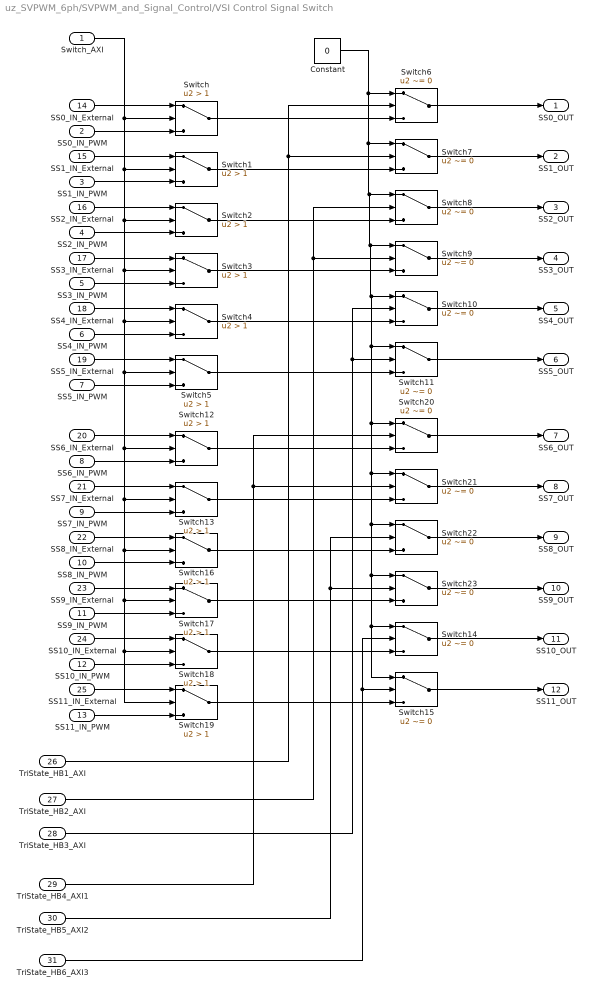
== system uz_SVPWM_6ph/SVPWM_and_Signal_Control/VSI Control Signal Switch ==
  Switch_AXI : Inport
  SS0_IN_PWM : Inport  Port=2
  SS1_IN_PWM : Inport  Port=3
  SS2_IN_PWM : Inport  Port=4
  SS3_IN_PWM : Inport  Port=5
  SS4_IN_PWM : Inport  Port=6
  SS5_IN_PWM : Inport  Port=7
  SS6_IN_PWM : Inport  Port=8
  SS7_IN_PWM : Inport  Port=9
  SS8_IN_PWM : Inport  Port=10
  SS9_IN_PWM : Inport  Port=11
  SS10_IN_PWM : Inport  Port=12
  SS11_IN_PWM : Inport  Port=13
  SS0_IN_External : Inport  Port=14
  SS1_IN_External : Inport  Port=15
  SS2_IN_External : Inport  Port=16
  SS3_IN_External : Inport  Port=17
  SS4_IN_External : Inport  Port=18
  SS5_IN_External : Inport  Port=19
  SS6_IN_External : Inport  Port=20
  SS7_IN_External : Inport  Port=21
  SS8_IN_External : Inport  Port=22
  SS9_IN_External : Inport  Port=23
  SS10_IN_External : Inport  Port=24
  SS11_IN_External : Inport  Port=25
  TriState_HB1_AXI : Inport  Port=26
  TriState_HB2_AXI : Inport  Port=27
  TriState_HB3_AXI : Inport  Port=28
  TriState_HB4_AXI1 : Inport  Port=29
  TriState_HB5_AXI2 : Inport  Port=30
  TriState_HB6_AXI3 : Inport  Port=31
  Constant : Constant  Value=0  OutDataTypeStr=boolean  SampleTime=T_FPGA_clk
  Switch{,1..5,12..13,16..19} (12 alike) : Switch  Criteria=u2 > Threshold  Threshold=1  SaturateOnIntegerOverflow=off  InputSameDT=off
  Switch{6..11,14..15,20..23} (12 alike) : Switch  Criteria=u2 ~= 0  Threshold=1  SaturateOnIntegerOverflow=off  InputSameDT=off
  SS0_OUT : Outport  VectorParamsAs1DForOutWhenUnconnected=off
  SS1_OUT : Outport  Port=2  VectorParamsAs1DForOutWhenUnconnected=off
  SS2_OUT : Outport  Port=3  VectorParamsAs1DForOutWhenUnconnected=off
  SS3_OUT : Outport  Port=4  VectorParamsAs1DForOutWhenUnconnected=off
  SS4_OUT : Outport  Port=5  VectorParamsAs1DForOutWhenUnconnected=off
  SS5_OUT : Outport  Port=6  VectorParamsAs1DForOutWhenUnconnected=off
  SS6_OUT : Outport  Port=7  VectorParamsAs1DForOutWhenUnconnected=off
  SS7_OUT : Outport  Port=8  VectorParamsAs1DForOutWhenUnconnected=off
  SS8_OUT : Outport  Port=9  VectorParamsAs1DForOutWhenUnconnected=off
  SS9_OUT : Outport  Port=10  VectorParamsAs1DForOutWhenUnconnected=off
  SS10_OUT : Outport  Port=11  VectorParamsAs1DForOutWhenUnconnected=off
  SS11_OUT : Outport  Port=12  VectorParamsAs1DForOutWhenUnconnected=off
  wires:
  Switch5/1 -> Switch11/3
  Switch/1 -> Switch6/3
  Switch3/1 -> Switch9/3
  Switch2/1 -> Switch8/3
  Switch1/1 -> Switch7/3
  Switch4/1 -> Switch10/3
  SS0_IN_PWM/1 -> Switch/3
  SS0_IN_External/1 -> Switch/1
  SS1_IN_External/1 -> Switch1/1
  SS1_IN_PWM/1 -> Switch1/3
  SS2_IN_External/1 -> Switch2/1
  SS2_IN_PWM/1 -> Switch2/3
  SS3_IN_External/1 -> Switch3/1
  SS3_IN_PWM/1 -> Switch3/3
  SS4_IN_External/1 -> Switch4/1
  SS4_IN_PWM/1 -> Switch4/3
  SS5_IN_External/1 -> Switch5/1
  SS5_IN_PWM/1 -> Switch5/3
  TriState_HB3_AXI/1 -> Switch10/2, Switch11/2
  TriState_HB2_AXI/1 -> Switch8/2, Switch9/2
  TriState_HB1_AXI/1 -> Switch6/2, Switch7/2
  Switch11/1 -> SS5_OUT/1
  Switch10/1 -> SS4_OUT/1
  Switch9/1 -> SS3_OUT/1
  Switch8/1 -> SS2_OUT/1
  Switch7/1 -> SS1_OUT/1
  Switch6/1 -> SS0_OUT/1
  Constant/1 -> Switch11/1, Switch20/1, Switch21/1, Switch14/1, Switch15/1, Switch23/1, Switch22/1, Switch10/1, Switch9/1, Switch8/1, Switch7/1, Switch6/1
  Switch20/1 -> SS6_OUT/1
  Switch21/1 -> SS7_OUT/1
  Switch22/1 -> SS8_OUT/1
  Switch23/1 -> SS9_OUT/1
  Switch14/1 -> SS10_OUT/1
  Switch15/1 -> SS11_OUT/1
  TriState_HB4_AXI1/1 -> Switch21/2, Switch20/2
  TriState_HB5_AXI2/1 -> Switch22/2, Switch23/2
  TriState_HB6_AXI3/1 -> Switch14/2, Switch15/2
  SS11_IN_PWM/1 -> Switch19/3
  SS11_IN_External/1 -> Switch19/1
  SS10_IN_PWM/1 -> Switch18/3
  SS10_IN_External/1 -> Switch18/1
  SS9_IN_PWM/1 -> Switch17/3
  SS9_IN_External/1 -> Switch17/1
  SS8_IN_PWM/1 -> Switch16/3
  SS8_IN_External/1 -> Switch16/1
  SS7_IN_PWM/1 -> Switch13/3
  SS7_IN_External/1 -> Switch13/1
  SS6_IN_External/1 -> Switch12/1
  SS6_IN_PWM/1 -> Switch12/3
  Switch18/1 -> Switch14/3
  Switch13/1 -> Switch21/3
  Switch16/1 -> Switch22/3
  Switch17/1 -> Switch23/3
  Switch12/1 -> Switch20/3
  Switch19/1 -> Switch15/3
  Switch_AXI/1 -> Switch12/2, Switch13/2, Switch16/2, Switch17/2, Switch19/2, Switch18/2, Switch5/2, Switch4/2, Switch3/2, Switch2/2, Switch1/2, Switch/2

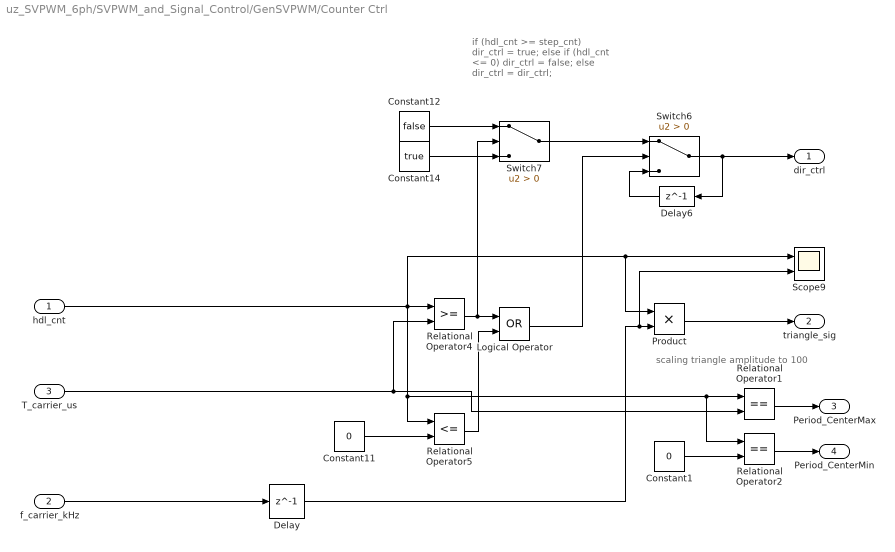
== system uz_SVPWM_6ph/SVPWM_and_Signal_Control/GenSVPWM/Counter Ctrl ==
  note: if (hdl_cnt >= step_cnt)
      | 	dir_ctrl = true;
      | else if (hdl_cnt <= 0)
      | 	dir_ctrl = false;
      | else
      | 	dir_ctrl = dir_ctrl;
  note: scaling triangle amplitude to 100
  hdl_cnt : Inport
  f_carrier_kHz : Inport  Port=2
  T_carrier_us : Inport  Port=3
  Constant1 : Constant  Value=0  OutDataTypeStr=fixdt(0,20,0)  SampleTime=T_FPGA_clk
  Constant11 : Constant  Value=0  OutDataTypeStr=fixdt(0,20,0)  SampleTime=T_FPGA_clk
  Constant12 : Constant  Value=false  SampleTime=T_FPGA_clk
  Constant14 : Constant  Value=true  SampleTime=T_FPGA_clk
  Delay : Delay  DelayLength=1
  Delay6 : Delay  DelayLength=1
  Logical Operator : Logic  Operator=OR  AllPortsSameDT=off  OutDataTypeStr=boolean
  Product : Product  OutDataTypeStr=fixdt(0,18,17)
  Relational Operator1 : RelationalOperator  Operator===  OutDataTypeStr=boolean  InputSameDT=off
  Relational Operator2 : RelationalOperator  Operator===  OutDataTypeStr=boolean  InputSameDT=off
  Relational Operator4 : RelationalOperator  OutDataTypeStr=boolean  InputSameDT=off
  Relational Operator5 : RelationalOperator  Operator=<=  OutDataTypeStr=boolean  InputSameDT=off
  Scope9 : Scope  NumInputPorts=2
  Switch6 : Switch  Criteria=u2 > Threshold  SaturateOnIntegerOverflow=off  InputSameDT=off
  Switch7 : Switch  Criteria=u2 > Threshold  SaturateOnIntegerOverflow=off  InputSameDT=off
  dir_ctrl : Outport  VectorParamsAs1DForOutWhenUnconnected=off
  triangle_sig : Outport  Port=2  VectorParamsAs1DForOutWhenUnconnected=off
  Period_CenterMax : Outport  Port=3  VectorParamsAs1DForOutWhenUnconnected=off
  Period_CenterMin : Outport  Port=4  VectorParamsAs1DForOutWhenUnconnected=off
  wires:
  hdl_cnt/1 -> Relational Operator2/1, Relational Operator1/1, Relational Operator5/1, Relational Operator4/1, Product/1, Scope9/1
  Switch6/1 -> Delay6/1, dir_ctrl/1
  Relational Operator4/1 -> Switch7/2, Logical Operator/1
  Relational Operator5/1 -> Logical Operator/2
  Constant11/1 -> Relational Operator5/2
  Logical Operator/1 -> Switch6/2
  Switch7/1 -> Switch6/1
  Constant12/1 -> Switch7/1
  Constant14/1 -> Switch7/3
  Delay6/1 -> Switch6/3
  T_carrier_us/1 -> Relational Operator4/2, Relational Operator1/2
  f_carrier_kHz/1 -> Delay/1
  Delay/1 -> Scope9/2, Product/2
  Relational Operator1/1 -> Period_CenterMax/1
  Relational Operator2/1 -> Period_CenterMin/1
  Constant1/1 -> Relational Operator2/2
  Product/1 -> triangle_sig/1

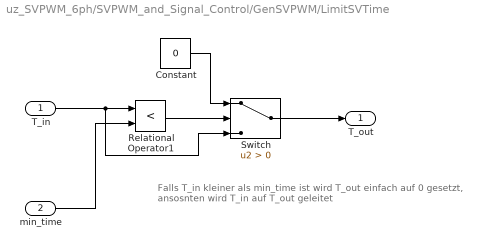
== system uz_SVPWM_6ph/SVPWM_and_Signal_Control/GenSVPWM/LimitSVTime ==
  note: Falls T_in kleiner als min_time ist wird T_out einfach auf 0 gesetzt,
      | ansosnten wird T_in auf T_out geleitet
  T_in : Inport
  min_time : Inport  Port=2
  Constant : Constant  Value=0  OutDataTypeStr=fixdt(1,18,16)  SampleTime=T_FPGA_clk
  Relational Operator1 : RelationalOperator  Operator=<  OutDataTypeStr=boolean  InputSameDT=off
  Switch : Switch  Criteria=u2 > Threshold  SaturateOnIntegerOverflow=off  InputSameDT=off
  T_out : Outport  VectorParamsAs1DForOutWhenUnconnected=off
  wires:
  min_time/1 -> Relational Operator1/2
  Switch/1 -> T_out/1
  T_in/1 -> Switch/3, Relational Operator1/1
  Relational Operator1/1 -> Switch/2
  Constant/1 -> Switch/1

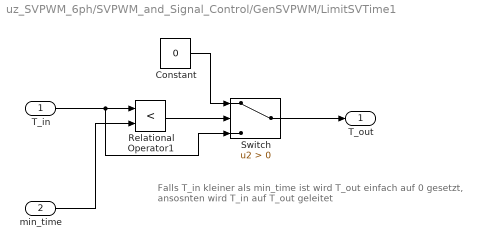
== system uz_SVPWM_6ph/SVPWM_and_Signal_Control/GenSVPWM/LimitSVTime1 ==
  note: Falls T_in kleiner als min_time ist wird T_out einfach auf 0 gesetzt,
      | ansosnten wird T_in auf T_out geleitet
  T_in : Inport
  min_time : Inport  Port=2
  Constant : Constant  Value=0  OutDataTypeStr=fixdt(1,18,16)  SampleTime=T_FPGA_clk
  Relational Operator1 : RelationalOperator  Operator=<  OutDataTypeStr=boolean  InputSameDT=off
  Switch : Switch  Criteria=u2 > Threshold  SaturateOnIntegerOverflow=off  InputSameDT=off
  T_out : Outport  VectorParamsAs1DForOutWhenUnconnected=off
  wires:
  Constant/1 -> Switch/1
  Relational Operator1/1 -> Switch/2
  T_in/1 -> Relational Operator1/1, Switch/3
  Switch/1 -> T_out/1
  min_time/1 -> Relational Operator1/2

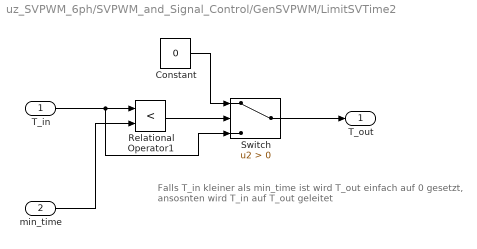
== system uz_SVPWM_6ph/SVPWM_and_Signal_Control/GenSVPWM/LimitSVTime2 ==
  note: Falls T_in kleiner als min_time ist wird T_out einfach auf 0 gesetzt,
      | ansosnten wird T_in auf T_out geleitet
  T_in : Inport
  min_time : Inport  Port=2
  Constant : Constant  Value=0  OutDataTypeStr=fixdt(1,18,16)  SampleTime=T_FPGA_clk
  Relational Operator1 : RelationalOperator  Operator=<  OutDataTypeStr=boolean  InputSameDT=off
  Switch : Switch  Criteria=u2 > Threshold  SaturateOnIntegerOverflow=off  InputSameDT=off
  T_out : Outport  VectorParamsAs1DForOutWhenUnconnected=off
  wires:
  min_time/1 -> Relational Operator1/2
  Switch/1 -> T_out/1
  T_in/1 -> Switch/3, Relational Operator1/1
  Relational Operator1/1 -> Switch/2
  Constant/1 -> Switch/1

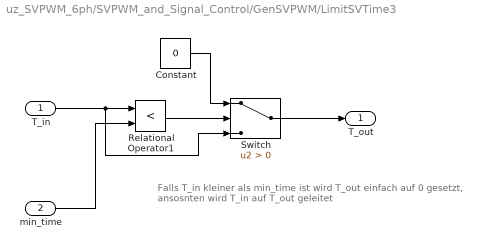
== system uz_SVPWM_6ph/SVPWM_and_Signal_Control/GenSVPWM/LimitSVTime3 ==
  note: Falls T_in kleiner als min_time ist wird T_out einfach auf 0 gesetzt,
      | ansosnten wird T_in auf T_out geleitet
  T_in : Inport
  min_time : Inport  Port=2
  Constant : Constant  Value=0  OutDataTypeStr=fixdt(1,18,16)  SampleTime=T_FPGA_clk
  Relational Operator1 : RelationalOperator  Operator=<  OutDataTypeStr=boolean  InputSameDT=off
  Switch : Switch  Criteria=u2 > Threshold  SaturateOnIntegerOverflow=off  InputSameDT=off
  T_out : Outport  VectorParamsAs1DForOutWhenUnconnected=off
  wires:
  Constant/1 -> Switch/1
  Relational Operator1/1 -> Switch/2
  T_in/1 -> Relational Operator1/1, Switch/3
  Switch/1 -> T_out/1
  min_time/1 -> Relational Operator1/2

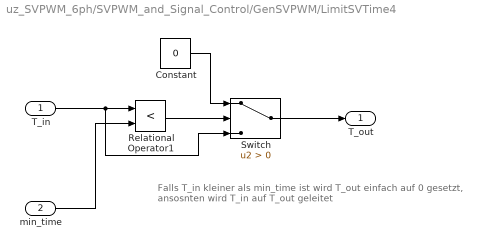
== system uz_SVPWM_6ph/SVPWM_and_Signal_Control/GenSVPWM/LimitSVTime4 ==
  note: Falls T_in kleiner als min_time ist wird T_out einfach auf 0 gesetzt,
      | ansosnten wird T_in auf T_out geleitet
  T_in : Inport
  min_time : Inport  Port=2
  Constant : Constant  Value=0  OutDataTypeStr=fixdt(1,18,16)  SampleTime=T_FPGA_clk
  Relational Operator1 : RelationalOperator  Operator=<  OutDataTypeStr=boolean  InputSameDT=off
  Switch : Switch  Criteria=u2 > Threshold  SaturateOnIntegerOverflow=off  InputSameDT=off
  T_out : Outport  VectorParamsAs1DForOutWhenUnconnected=off
  wires:
  min_time/1 -> Relational Operator1/2
  Switch/1 -> T_out/1
  T_in/1 -> Switch/3, Relational Operator1/1
  Relational Operator1/1 -> Switch/2
  Constant/1 -> Switch/1
